simulink subsystem "DynamicSteering"  (R2023b)
settings: Solver=VariableStepAuto  StartTime=0.0  StopTime=10.0  RelTol=1e-3
undefined symbols (not defined in the file): PlntSteerRatio, PlntVehDstCGFrntAxl, PlntVehDstCGRearAxl, PlntVehTrckWdth
libraries: vehdynlibsteering x2
settings Model: ModifiedByFormat=The MathWorks, Inc.  Creator=The MathWorks, Inc.  LastModifiedBy=The MathWorks, Inc.

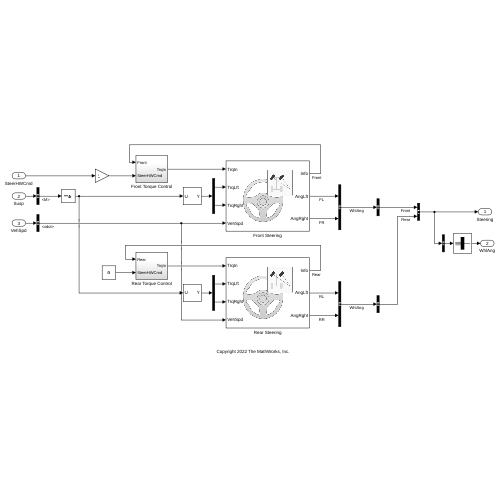
[thumbnail: Simulink's stored preview of the top-level diagram]
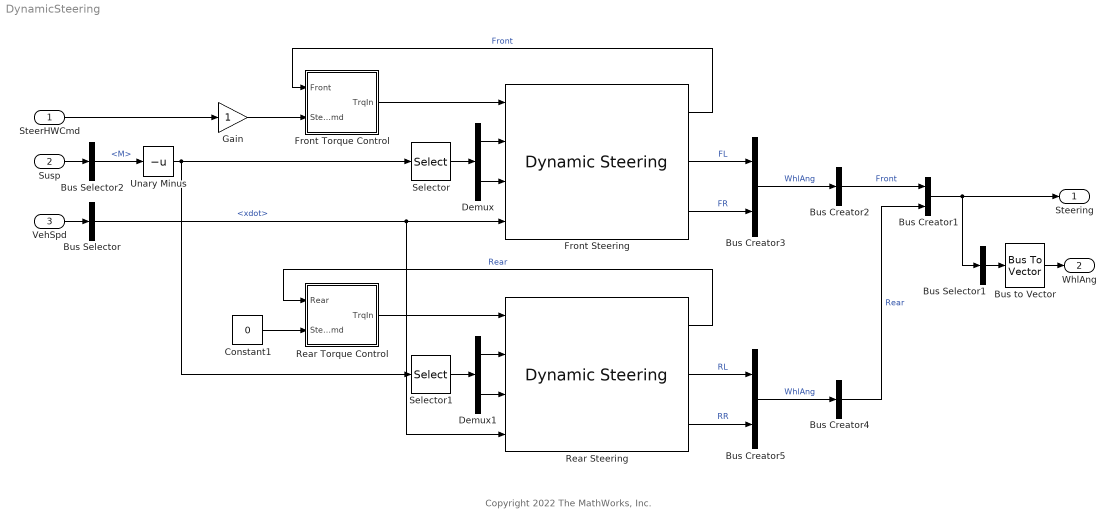
== system DynamicSteering ==
  note: Copyright 2022 The MathWorks, Inc.
  SteerHWCmd : Inport
  Susp : Inport  Port=2
  VehSpd : Inport  Port=3
  Bus Creator1 : BusCreator  Inputs=2
  Bus Creator2 : BusCreator  Inputs=1
  Bus Creator3 : BusCreator  Inputs=2
  Bus Creator4 : BusCreator  Inputs=1
  Bus Creator5 : BusCreator  Inputs=2
  Bus Selector : BusSelector  OutputSignals=BdyFrm.Cg.Vel.xdot
  Bus Selector1 : BusSelector  OutputSignals=Front.WhlAng.FL,Front.WhlAng.FR,Rear.WhlAng.RL,Rear.WhlAng.RR  OutputAsBus=on
  Bus Selector2 : BusSelector  OutputSignals=SuspChassis.Veh.M
  Bus to Vector : BusToVector
  Constant1 : Constant  Value=0  SampleTime=-1
  Demux : Demux  Outputs=2
  Demux1 : Demux  Outputs=2
  Front Steering : vehdynlibsteering/Dynamic Steering  StrgType=Ackerman  StrgRatioType=Constant  PwrAst=on  Loc=Front  TrckWdth=PlntVehTrckWdth(1)  WhlBase=PlntVehDstCGFrntAxl+PlntVehDstCGRearAxl  StrgRng=PlntSteerRange  StrgAngBpts="[-6.2832   -5.0265   -3.7699   -2.5133   -1.2566         0    1.2566    2.5133    3.7699    5.0265    6.2832]"  StrgRatioTbl=|  StrgRatio=PlntSteerRatio  StrgArmLngth=0.1  RckCsLngth=0.5  TieRodLngth=0.248  D=0.2  PnnRadiusTbl="[0.0055    0.0055    0.0056    0.0057    0.0057    0.0057    0.0058    0.0057    0.0056    0.0055    0.0055]"  PnnRadius=0.0057  RodLngth=0.1  ParaArmLngth=0.9  J1=PlntSteerUpperInertia  J2=PlntSteerLowerInertia  beta_u=0.1  beta_l=0.1  b1=0.001  k1=PlntSteerHysStiff  b2=1  b3=0.001  theta_o=0  omega_o=0  FricTrq=0  TrqBpts=PlntSteerWheelTrqBpt  VehSpdBpts=[0 20]  TrqTbl=PlntSteerTrqAsstTbl  TrqLmt=PlntSteerTrqLimit  PwrLmt=PlntSteerPwrLimit  Eta=1  omega_c=PlntSteerWc  aMode=2
      | [13.5000   13.3750   13.2500   13.1250   13.0000   13.0000   13.0000   13.1250   13.2500   13.3750   13.5000
      | ]
  Front Torque Control : Subsystem
  Gain : Gain
  Rear Steering : vehdynlibsteering/Dynamic Steering  StrgType=Ackerman  StrgRatioType=Constant  PwrAst=on  Loc=Rear  TrckWdth=PlntVehTrckWdth(1)  WhlBase=PlntVehDstCGFrntAxl+PlntVehDstCGRearAxl  StrgRng=PlntSteerRange  StrgAngBpts="[-6.2832   -5.0265   -3.7699   -2.5133   -1.2566         0    1.2566    2.5133    3.7699    5.0265    6.2832]"  StrgRatioTbl=|  StrgRatio=PlntSteerRatio*10  StrgArmLngth=0.1  RckCsLngth=0.5  TieRodLngth=0.248  D=0.2  PnnRadiusTbl="[0.0055    0.0055    0.0056    0.0057    0.0057    0.0057    0.0058    0.0057    0.0056    0.0055    0.0055]"  PnnRadius=0.0057  RodLngth=0.1  ParaArmLngth=0.9  J1=PlntSteerUpperInertia  J2=PlntSteerLowerInertia  beta_u=0.1  beta_l=0.1  b1=0.001  k1=PlntSteerHysStiff  b2=1  b3=0.001  theta_o=0  omega_o=0  FricTrq=0  TrqBpts=PlntSteerWheelTrqBpt  VehSpdBpts=[0 20]  TrqTbl=PlntSteerTrqAsstTbl  TrqLmt=PlntSteerTrqLimit  PwrLmt=PlntSteerPwrLimit  Eta=1  omega_c=PlntSteerWc  aMode=2
      | [13.5000   13.3750   13.2500   13.1250   13.0000   13.0000   13.0000   13.1250   13.2500   13.3750   13.5000
      | ]
  Rear Torque Control : Subsystem
  Selector : Selector  NumberOfDimensions=2  InputPortWidth=3  IndexOptions=Index vector (dialog),Index vector (dialog)  Indices=[3],[1 2]  OutputSizes=1,1
  Selector1 : Selector  NumberOfDimensions=2  InputPortWidth=3  IndexOptions=Index vector (dialog),Index vector (dialog)  Indices=[3],[1 2]  OutputSizes=1,1
  Unary Minus : UnaryMinus
  Steering : Outport
  WhlAng : Outport  Port=2  Unit=rad  VectorParamsAs1DForOutWhenUnconnected=off
  wires:
  Front Torque Control/1(TrqIn) -> Front Steering/1
  Front Steering/1 -> Front Torque Control/1(Front)  "Front"
  SteerHWCmd/1 -> Gain/1
  Demux1/2 -> Rear Steering/3
  Bus Selector2/1 -> Unary Minus/1  "<M>"
  Demux1/1 -> Rear Steering/2
  Selector1/1 -> Demux1/1
  Selector/1 -> Demux/1
  Demux/2 -> Front Steering/3
  Demux/1 -> Front Steering/2
  VehSpd/1 -> Bus Selector/1
  Bus Selector/1 -> Rear Steering/4, Front Steering/4  "<xdot>"
  Susp/1 -> Bus Selector2/1
  Rear Torque Control/1(TrqIn) -> Rear Steering/1
  Bus Creator3/1 -> Bus Creator2/1  "WhlAng"
  Bus Creator4/1 -> Bus Creator1/2  "Rear"
  Front Steering/2 -> Bus Creator3/1  "FL"
  Rear Steering/2 -> Bus Creator5/1  "RL"
  Rear Steering/3 -> Bus Creator5/2  "RR"
  Bus Creator2/1 -> Bus Creator1/1  "Front"
  Front Steering/3 -> Bus Creator3/2  "FR"
  Bus Creator5/1 -> Bus Creator4/1  "WhlAng"
  Rear Steering/1 -> Rear Torque Control/1(Rear)  "Rear"
  Bus Selector1/1 -> Bus to Vector/1
  Bus Creator1/1 -> Steering/1, Bus Selector1/1
  Bus to Vector/1 -> WhlAng/1
  Constant1/1 -> Rear Torque Control/2(SteerHWCmd)
  Unary Minus/1 -> Selector1/1, Selector/1
  Gain/1 -> Front Torque Control/2(SteerHWCmd)

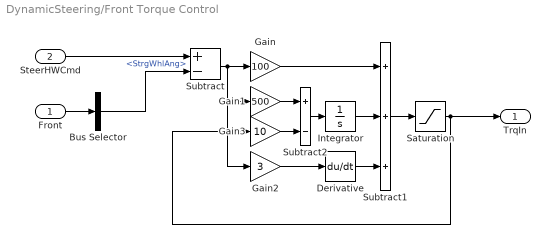
== system DynamicSteering/Front Torque Control ==
  Front : Inport
  SteerHWCmd : Inport  Port=2
  Bus Selector : BusSelector  OutputSignals=StrgWhlAng
  Derivative : Derivative  CoefficientInTFapproximation=1000
  Gain : Gain  Gain=100
  Gain1 : Gain  Gain=500
  Gain2 : Gain  Gain=3
  Gain3 : Gain  Gain=10
  Integrator : Integrator  LimitOutput=on  UpperSaturationLimit=50  LowerSaturationLimit=-50
  Saturation : Saturate  UpperLimit=500  LowerLimit=-500
  Subtract : Sum  Inputs=+-
  Subtract1 : Sum  Inputs=+++
  Subtract2 : Sum  Inputs=+-
  TrqIn : Outport
  wires:
  Front/1 -> Bus Selector/1
  Gain/1 -> Subtract1/1
  Saturation/1 -> TrqIn/1, Gain3/1
  Subtract2/1 -> Integrator/1
  Gain2/1 -> Derivative/1
  Gain1/1 -> Subtract2/1
  Gain3/1 -> Subtract2/2
  Subtract/1 -> Gain2/1, Gain1/1, Gain/1
  Integrator/1 -> Subtract1/2
  Derivative/1 -> Subtract1/3
  Bus Selector/1 -> Subtract/2  "<StrgWhlAng>"
  Subtract1/1 -> Saturation/1
  SteerHWCmd/1 -> Subtract/1

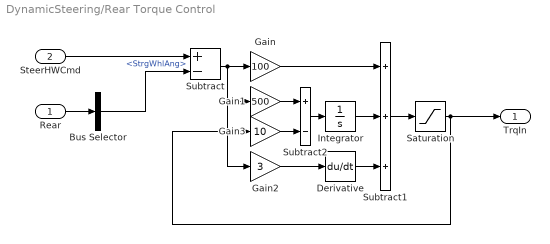
== system DynamicSteering/Rear Torque Control ==
  Rear : Inport
  SteerHWCmd : Inport  Port=2
  Bus Selector : BusSelector  OutputSignals=StrgWhlAng
  Derivative : Derivative  CoefficientInTFapproximation=1000
  Gain : Gain  Gain=100
  Gain1 : Gain  Gain=500
  Gain2 : Gain  Gain=3
  Gain3 : Gain  Gain=10
  Integrator : Integrator  LimitOutput=on  UpperSaturationLimit=50  LowerSaturationLimit=-50
  Saturation : Saturate  UpperLimit=500  LowerLimit=-500
  Subtract : Sum  Inputs=+-
  Subtract1 : Sum  Inputs=+++
  Subtract2 : Sum  Inputs=+-
  TrqIn : Outport
  wires:
  SteerHWCmd/1 -> Subtract/1
  Subtract1/1 -> Saturation/1
  Bus Selector/1 -> Subtract/2  "<StrgWhlAng>"
  Derivative/1 -> Subtract1/3
  Integrator/1 -> Subtract1/2
  Subtract/1 -> Gain/1, Gain1/1, Gain2/1
  Gain3/1 -> Subtract2/2
  Gain1/1 -> Subtract2/1
  Gain2/1 -> Derivative/1
  Subtract2/1 -> Integrator/1
  Saturation/1 -> Gain3/1, TrqIn/1
  Gain/1 -> Subtract1/1
  Rear/1 -> Bus Selector/1
